simulink model "TirePressureSignalLogic"  (R2025b)
settings: Solver=VariableStepAuto  StartTime=0.0  StopTime=10  RelTol=1e-3
undefined symbols (not defined in the file): DiscIntNeverNeededParam
settings Model: Creator=kimsv  LastModifiedBy=kimsv

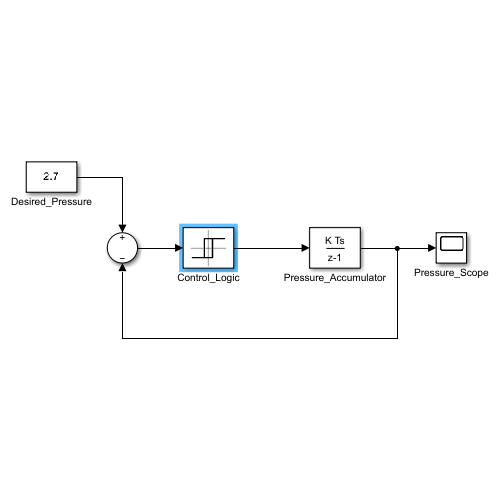
[thumbnail: Simulink's stored preview of the top-level diagram]
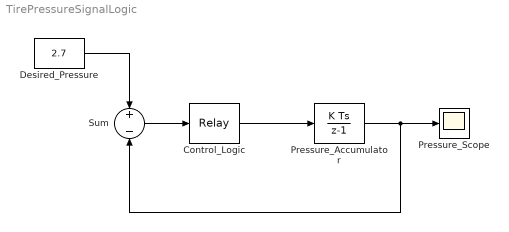
== system TirePressureSignalLogic ==
  Control_Logic : Relay  OnSwitchValue=2  OffSwitchValue=0  OnOutputValue=0.5
  Desired_Pressure : Constant  Value=2.7
  Pressure_Accumulator : DiscreteIntegrator  InitialCondition=2  SampleTime=0.1  ICPrevOutput=DiscIntNeverNeededParam  ICPrevScaledInput=DiscIntNeverNeededParam
  Pressure_Scope : Scope
      settings: ActiveDisplayYMinimum=1  ActiveDisplayYMaximum=3
  Sum : Sum  Inputs=+-
  wires:
  Desired_Pressure/1 -> Sum/1
  Sum/1 -> Control_Logic/1
  Control_Logic/1 -> Pressure_Accumulator/1
  Pressure_Accumulator/1 -> Pressure_Scope/1, Sum/2
